simulink model "2_RLC_S"  (R2024b)
settings: Solver=VariableStepAuto  StartTime=0.0  StopTime=0.0001  MaxStep=0.0000001  RelTol=1e-3
InitFcn:
  | R = 120;
  | L = 0.0004;
  | C = 0.0000001;
  | V_in = 1;

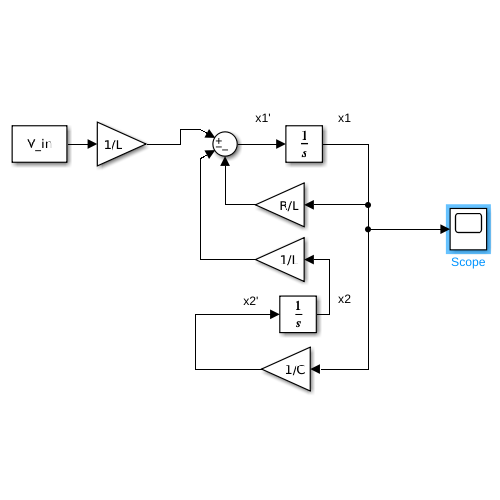
[thumbnail: Simulink's stored preview of the top-level diagram]
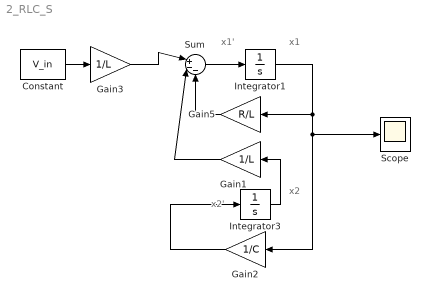
== system 2_RLC_S ==
  note: x2'
  note: x1'
  note: x1
  note: x2
  Constant : Constant  Value=V_in
  Gain1 : Gain  Gain=1/L
  Gain2 : Gain  Gain=1/C
  Gain3 : Gain  Gain=1/L
  Gain5 : Gain  Gain=R/L
  Integrator1 : Integrator
  Integrator3 : Integrator
  Scope : Scope
  Sum : Sum  Inputs=|+--
  wires:
  Integrator1/1 -> Gain5/1, Gain2/1, Scope/1
  Sum/1 -> Integrator1/1
  Constant/1 -> Gain3/1
  Integrator3/1 -> Gain1/1
  Gain2/1 -> Integrator3/1
  Gain3/1 -> Sum/1
  Gain1/1 -> Sum/2
  Gain5/1 -> Sum/3
